simulink subsystem "Encoders"  (R2023a)
settings: Solver=VariableStepAuto  StartTime=0.0  StopTime=10.0  RelTol=1e-3
libraries: dspswit3 x2
settings Model: Creator=JesseJabezArendse  LastModifiedBy=JesseJabezArendse

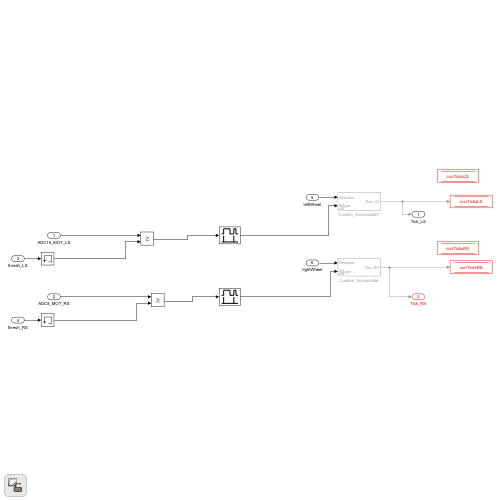
[thumbnail: Simulink's stored preview of the top-level diagram]
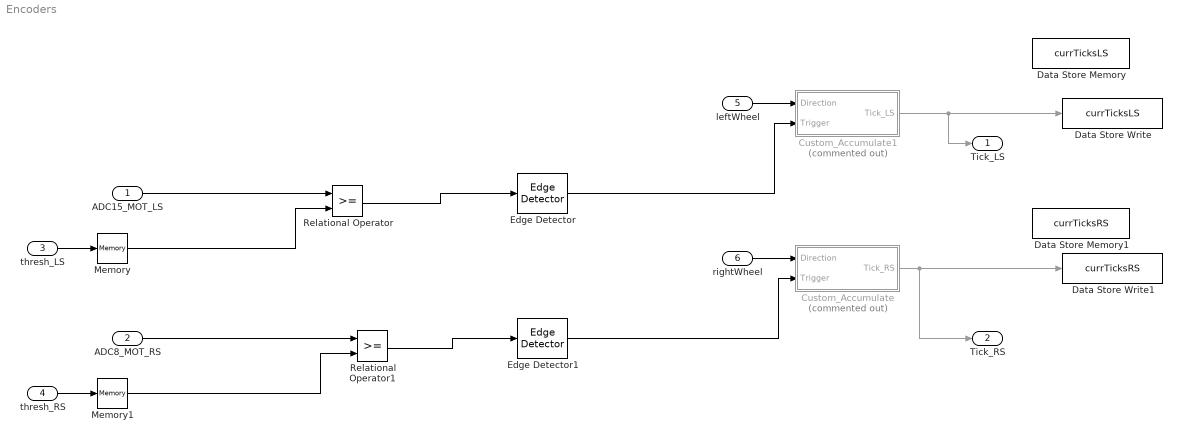
== system Encoders ==
  ADC15_MOT_LS : Inport
  ADC8_MOT_RS : Inport  Port=2
  thresh_LS : Inport  Port=3  OutDataTypeStr=uint16  PortDimensions=1
  thresh_RS : Inport  Port=4  OutDataTypeStr=uint16  PortDimensions=1
  leftWheel : Inport  Port=5
  rightWheel : Inport  Port=6
  Custom_Accumulate : Subsystem  Commented=on
  Custom_Accumulate1 : Subsystem  Commented=on
  Data Store Memory : DataStoreMemory  DataStoreName=currTicksLS  WriteAfterWriteMsg=warning  ShowAdditionalParam=off  OutDataTypeStr=uint32  Dimensions=1
  Data Store Memory1 : DataStoreMemory  DataStoreName=currTicksRS  WriteAfterWriteMsg=warning  ShowAdditionalParam=off  OutDataTypeStr=uint32  Dimensions=1
  Data Store Write : DataStoreWrite  DataStoreName=currTicksLS  IndexOptions=Index vector (dialog)  Indices=1  OutputSizes=1
  Data Store Write1 : DataStoreWrite  DataStoreName=currTicksRS  IndexOptions=Index vector (dialog)  Indices=1  OutputSizes=1
  Edge Detector : dspswit3/Edge Detector  InputProcessing=Columns as channels (frame based)
  Edge Detector1 : dspswit3/Edge Detector  InputProcessing=Columns as channels (frame based)
  Memory : Memory  InheritSampleTime=on
  Memory1 : Memory  InheritSampleTime=on
  Relational Operator : RelationalOperator  OutDataTypeStr=boolean  RndMeth=Simplest  InputSameDT=off
  Relational Operator1 : RelationalOperator  OutDataTypeStr=boolean  RndMeth=Simplest  InputSameDT=off
  Tick_LS : Outport  OutDataTypeStr=uint32  PortDimensions=1
  Tick_RS : Outport  Port=2  OutDataTypeStr=uint32  PortDimensions=1
  wires:
  ADC15_MOT_LS/1 -> Relational Operator/1
  thresh_LS/1 -> Memory/1
  thresh_RS/1 -> Memory1/1
  Memory/1 -> Relational Operator/2
  Relational Operator/1 -> Edge Detector/1
  Edge Detector/1 -> Custom_Accumulate1/2(Trigger)
  Memory1/1 -> Relational Operator1/2
  Relational Operator1/1 -> Edge Detector1/1
  ADC8_MOT_RS/1 -> Relational Operator1/1
  leftWheel/1 -> Custom_Accumulate1/1(Direction)
  Custom_Accumulate1/1(Tick_LS) -> Tick_LS/1, Data Store Write/1
  rightWheel/1 -> Custom_Accumulate/1(Direction)
  Edge Detector1/1 -> Custom_Accumulate/2(Trigger)
  Custom_Accumulate/1(Tick_RS) -> Data Store Write1/1, Tick_RS/1

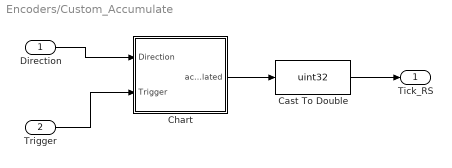
== system Encoders/Custom_Accumulate ==
  Direction : Inport
  Trigger : Inport  Port=2
  Cast To Double : DataTypeConversion  OutDataTypeStr=uint32  SaturateOnIntegerOverflow=off  RndMeth=Floor
  Chart : Stateflow chart  TreatAsAtomicUnit=on
  Tick_RS : Outport
  wires:
  Direction/1 -> Chart/1(Direction)
  Chart/1(accumulated) -> Cast To Double/1
  Trigger/1 -> Chart/2(Trigger)
  Cast To Double/1 -> Tick_RS/1

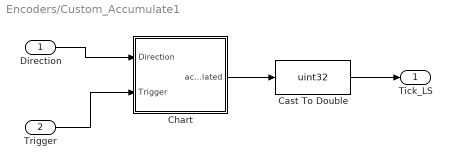
== system Encoders/Custom_Accumulate1 ==
  Direction : Inport
  Trigger : Inport  Port=2
  Cast To Double : DataTypeConversion  OutDataTypeStr=uint32  SaturateOnIntegerOverflow=off  RndMeth=Floor
  Chart : Stateflow chart  TreatAsAtomicUnit=on
  Tick_LS : Outport
  wires:
  Direction/1 -> Chart/1(Direction)
  Chart/1(accumulated) -> Cast To Double/1
  Trigger/1 -> Chart/2(Trigger)
  Cast To Double/1 -> Tick_LS/1

== stateflow chart Encoders/Custom_Accumulate/Chart ==
  state Accum
    state back
      entry:
      accumulated = accumulated - 1;
    state foward
      entry:
      accumulated = accumulated + 1;
    Accum -> foward [order 1] : [Trigger == 1 && Direction > 0]
    (default) -> foward
    Accum -> back [order 2] : [Trigger == 1 && Direction < 0]
  (default) -> Accum
  data: Direction input; Trigger input; accumulated output =0

== stateflow chart Encoders/Custom_Accumulate1/Chart ==
  state Accum
    state back
      entry:
      accumulated = accumulated - 1;
    state foward
      entry:
      accumulated = accumulated + 1;
    Accum -> foward [order 1] : [Trigger == 1 && Direction > 0]
    (default) -> foward
    Accum -> back [order 2] : [Trigger == 1 && Direction < 0]
  (default) -> Accum
  data: Direction input; Trigger input; accumulated output =0
